simulink model "QuadRotor2Arm"  (R2019b)
(part 3 of 15)

  Revolute64 : sm_lib/Joints/Revolute Joint  JointMode=Normal  SenseConstraintForce=off  SenseConstraintForceX=off  SenseConstraintForceY=off  SenseConstraintForceZ=off  SenseConstraintTorque=off  SenseConstraintTorqueX=off  SenseConstraintTorqueY=off  SenseConstraintTorqueZ=off  SenseTotalForce=off  SenseTotalForceX=off  SenseTotalForceY=off  SenseTotalForceZ=off  SenseTotalTorque=off  SenseTotalTorqueX=off  SenseTotalTorqueY=off  SenseTotalTorqueZ=off  CompositeWrenchDir=FollowerOnBase  CompositeWrenchFrame=BaseFrame  EquilibriumPosition=0  EquilibriumPositionUnits=rad  SpringStiffness=0  SpringStiffnessUnits=N*m/rad  DampingCoefficient=0  DampingCoefficientUnits=N*m/(rad/s)  TorqueActuationMode=NoTorque  MotionActuationMode=ComputedMotion  SensePosition=off  SenseVelocity=off  SenseAcceleration=off  SenseTorqueForce=off  SenseLowerLimitTorqueForce=off  SenseUpperLimitTorqueForce=off  LowerLimitSpecify=off  LowerLimitBound=-90  LowerLimitBoundUnits=deg  LowerLimitStiffness=1e4  LowerLimitStiffnessUnits=N*m/deg  LowerLimitDamping=10  LowerLimitDampingUnits=N*m/(deg/s)  LowerLimitTransitionRegionWidth=0.1  LowerLimitTransitionRegionWidthUnits=deg  UpperLimitSpecify=off  UpperLimitBound=90  UpperLimitBoundUnits=deg  UpperLimitStiffness=1e4  UpperLimitStiffnessUnits=N*m/deg  UpperLimitDamping=10  UpperLimitDampingUnits=N*m/(deg/s)  UpperLimitTransitionRegionWidth=0.1  UpperLimitTransitionRegionWidthUnits=deg  PositionTargetSpecify=on  PositionTargetPriority=Low  PositionTargetValue=smiData.RevoluteJoint(65).Rz.Pos  PositionTargetValueUnits=deg  VelocityTargetSpecify=off  VelocityTargetPriority=High  VelocityTargetValue=0  VelocityTargetValueUnits=deg/s
  Revolute65 : sm_lib/Joints/Revolute Joint  JointMode=Normal  SenseConstraintForce=off  SenseConstraintForceX=off  SenseConstraintForceY=off  SenseConstraintForceZ=off  SenseConstraintTorque=off  SenseConstraintTorqueX=off  SenseConstraintTorqueY=off  SenseConstraintTorqueZ=off  SenseTotalForce=off  SenseTotalForceX=off  SenseTotalForceY=off  SenseTotalForceZ=off  SenseTotalTorque=off  SenseTotalTorqueX=off  SenseTotalTorqueY=off  SenseTotalTorqueZ=off  CompositeWrenchDir=FollowerOnBase  CompositeWrenchFrame=BaseFrame  EquilibriumPosition=0  EquilibriumPositionUnits=rad  SpringStiffness=0  SpringStiffnessUnits=N*m/rad  DampingCoefficient=0  DampingCoefficientUnits=N*m/(rad/s)  TorqueActuationMode=NoTorque  MotionActuationMode=ComputedMotion  SensePosition=off  SenseVelocity=off  SenseAcceleration=off  SenseTorqueForce=off  SenseLowerLimitTorqueForce=off  SenseUpperLimitTorqueForce=off  LowerLimitSpecify=off  LowerLimitBound=-90  LowerLimitBoundUnits=deg  LowerLimitStiffness=1e4  LowerLimitStiffnessUnits=N*m/deg  LowerLimitDamping=10  LowerLimitDampingUnits=N*m/(deg/s)  LowerLimitTransitionRegionWidth=0.1  LowerLimitTransitionRegionWidthUnits=deg  UpperLimitSpecify=off  UpperLimitBound=90  UpperLimitBoundUnits=deg  UpperLimitStiffness=1e4  UpperLimitStiffnessUnits=N*m/deg  UpperLimitDamping=10  UpperLimitDampingUnits=N*m/(deg/s)  UpperLimitTransitionRegionWidth=0.1  UpperLimitTransitionRegionWidthUnits=deg  PositionTargetSpecify=on  PositionTargetPriority=Low  PositionTargetValue=smiData.RevoluteJoint(66).Rz.Pos  PositionTargetValueUnits=deg  VelocityTargetSpecify=off  VelocityTargetPriority=High  VelocityTargetValue=0  VelocityTargetValueUnits=deg/s
  Revolute66 : sm_lib/Joints/Revolute Joint  JointMode=Normal  SenseConstraintForce=off  SenseConstraintForceX=off  SenseConstraintForceY=off  SenseConstraintForceZ=off  SenseConstraintTorque=off  SenseConstraintTorqueX=off  SenseConstraintTorqueY=off  SenseConstraintTorqueZ=off  SenseTotalForce=off  SenseTotalForceX=off  SenseTotalForceY=off  SenseTotalForceZ=off  SenseTotalTorque=off  SenseTotalTorqueX=off  SenseTotalTorqueY=off  SenseTotalTorqueZ=off  CompositeWrenchDir=FollowerOnBase  CompositeWrenchFrame=BaseFrame  EquilibriumPosition=0  EquilibriumPositionUnits=rad  SpringStiffness=0  SpringStiffnessUnits=N*m/rad  DampingCoefficient=0  DampingCoefficientUnits=N*m/(rad/s)  TorqueActuationMode=NoTorque  MotionActuationMode=ComputedMotion  SensePosition=off  SenseVelocity=off  SenseAcceleration=off  SenseTorqueForce=off  SenseLowerLimitTorqueForce=off  SenseUpperLimitTorqueForce=off  LowerLimitSpecify=off  LowerLimitBound=-90  LowerLimitBoundUnits=deg  LowerLimitStiffness=1e4  LowerLimitStiffnessUnits=N*m/deg  LowerLimitDamping=10  LowerLimitDampingUnits=N*m/(deg/s)  LowerLimitTransitionRegionWidth=0.1  LowerLimitTransitionRegionWidthUnits=deg  UpperLimitSpecify=off  UpperLimitBound=90  UpperLimitBoundUnits=deg  UpperLimitStiffness=1e4  UpperLimitStiffnessUnits=N*m/deg  UpperLimitDamping=10  UpperLimitDampingUnits=N*m/(deg/s)  UpperLimitTransitionRegionWidth=0.1  UpperLimitTransitionRegionWidthUnits=deg  PositionTargetSpecify=on  PositionTargetPriority=Low  PositionTargetValue=smiData.RevoluteJoint(67).Rz.Pos  PositionTargetValueUnits=deg  VelocityTargetSpecify=off  VelocityTargetPriority=High  VelocityTargetValue=0  VelocityTargetValueUnits=deg/s
  Revolute67 : sm_lib/Joints/Revolute Joint  JointMode=Normal  SenseConstraintForce=off  SenseConstraintForceX=off  SenseConstraintForceY=off  SenseConstraintForceZ=off  SenseConstraintTorque=off  SenseConstraintTorqueX=off  SenseConstraintTorqueY=off  SenseConstraintTorqueZ=off  SenseTotalForce=off  SenseTotalForceX=off  SenseTotalForceY=off  SenseTotalForceZ=off  SenseTotalTorque=off  SenseTotalTorqueX=off  SenseTotalTorqueY=off  SenseTotalTorqueZ=off  CompositeWrenchDir=FollowerOnBase  CompositeWrenchFrame=BaseFrame  EquilibriumPosition=0  EquilibriumPositionUnits=rad  SpringStiffness=0  SpringStiffnessUnits=N*m/rad  DampingCoefficient=0  DampingCoefficientUnits=N*m/(rad/s)  TorqueActuationMode=NoTorque  MotionActuationMode=ComputedMotion  SensePosition=off  SenseVelocity=off  SenseAcceleration=off  SenseTorqueForce=off  SenseLowerLimitTorqueForce=off  SenseUpperLimitTorqueForce=off  LowerLimitSpecify=off  LowerLimitBound=-90  LowerLimitBoundUnits=deg  LowerLimitStiffness=1e4  LowerLimitStiffnessUnits=N*m/deg  LowerLimitDamping=10  LowerLimitDampingUnits=N*m/(deg/s)  LowerLimitTransitionRegionWidth=0.1  LowerLimitTransitionRegionWidthUnits=deg  UpperLimitSpecify=off  UpperLimitBound=90  UpperLimitBoundUnits=deg  UpperLimitStiffness=1e4  UpperLimitStiffnessUnits=N*m/deg  UpperLimitDamping=10  UpperLimitDampingUnits=N*m/(deg/s)  UpperLimitTransitionRegionWidth=0.1  UpperLimitTransitionRegionWidthUnits=deg  PositionTargetSpecify=on  PositionTargetPriority=Low  PositionTargetValue=smiData.RevoluteJoint(68).Rz.Pos  PositionTargetValueUnits=deg  VelocityTargetSpecify=off  VelocityTargetPriority=High  VelocityTargetValue=0  VelocityTargetValueUnits=deg/s
  Revolute68 : sm_lib/Joints/Revolute Joint  JointMode=Normal  SenseConstraintForce=off  SenseConstraintForceX=off  SenseConstraintForceY=off  SenseConstraintForceZ=off  SenseConstraintTorque=off  SenseConstraintTorqueX=off  SenseConstraintTorqueY=off  SenseConstraintTorqueZ=off  SenseTotalForce=off  SenseTotalForceX=off  SenseTotalForceY=off  SenseTotalForceZ=off  SenseTotalTorque=off  SenseTotalTorqueX=off  SenseTotalTorqueY=off  SenseTotalTorqueZ=off  CompositeWrenchDir=FollowerOnBase  CompositeWrenchFrame=BaseFrame  EquilibriumPosition=0  EquilibriumPositionUnits=rad  SpringStiffness=0  SpringStiffnessUnits=N*m/rad  DampingCoefficient=0  DampingCoefficientUnits=N*m/(rad/s)  TorqueActuationMode=NoTorque  MotionActuationMode=ComputedMotion  SensePosition=off  SenseVelocity=off  SenseAcceleration=off  SenseTorqueForce=off  SenseLowerLimitTorqueForce=off  SenseUpperLimitTorqueForce=off  LowerLimitSpecify=off  LowerLimitBound=-90  LowerLimitBoundUnits=deg  LowerLimitStiffness=1e4  LowerLimitStiffnessUnits=N*m/deg  LowerLimitDamping=10  LowerLimitDampingUnits=N*m/(deg/s)  LowerLimitTransitionRegionWidth=0.1  LowerLimitTransitionRegionWidthUnits=deg  UpperLimitSpecify=off  UpperLimitBound=90  UpperLimitBoundUnits=deg  UpperLimitStiffness=1e4  UpperLimitStiffnessUnits=N*m/deg  UpperLimitDamping=10  UpperLimitDampingUnits=N*m/(deg/s)  UpperLimitTransitionRegionWidth=0.1  UpperLimitTransitionRegionWidthUnits=deg  PositionTargetSpecify=on  PositionTargetPriority=Low  PositionTargetValue=smiData.RevoluteJoint(69).Rz.Pos  PositionTargetValueUnits=deg  VelocityTargetSpecify=off  VelocityTargetPriority=High  VelocityTargetValue=0  VelocityTargetValueUnits=deg/s
  Revolute69 : sm_lib/Joints/Revolute Joint  JointMode=Normal  SenseConstraintForce=off  SenseConstraintForceX=off  SenseConstraintForceY=off  SenseConstraintForceZ=off  SenseConstraintTorque=off  SenseConstraintTorqueX=off  SenseConstraintTorqueY=off  SenseConstraintTorqueZ=off  SenseTotalForce=off  SenseTotalForceX=off  SenseTotalForceY=off  SenseTotalForceZ=off  SenseTotalTorque=off  SenseTotalTorqueX=off  SenseTotalTorqueY=off  SenseTotalTorqueZ=off  CompositeWrenchDir=FollowerOnBase  CompositeWrenchFrame=BaseFrame  EquilibriumPosition=0  EquilibriumPositionUnits=rad  SpringStiffness=0  SpringStiffnessUnits=N*m/rad  DampingCoefficient=0  DampingCoefficientUnits=N*m/(rad/s)  TorqueActuationMode=NoTorque  MotionActuationMode=ComputedMotion  SensePosition=off  SenseVelocity=off  SenseAcceleration=off  SenseTorqueForce=off  SenseLowerLimitTorqueForce=off  SenseUpperLimitTorqueForce=off  LowerLimitSpecify=off  LowerLimitBound=-90  LowerLimitBoundUnits=deg  LowerLimitStiffness=1e4  LowerLimitStiffnessUnits=N*m/deg  LowerLimitDamping=10  LowerLimitDampingUnits=N*m/(deg/s)  LowerLimitTransitionRegionWidth=0.1  LowerLimitTransitionRegionWidthUnits=deg  UpperLimitSpecify=off  UpperLimitBound=90  UpperLimitBoundUnits=deg  UpperLimitStiffness=1e4  UpperLimitStiffnessUnits=N*m/deg  UpperLimitDamping=10  UpperLimitDampingUnits=N*m/(deg/s)  UpperLimitTransitionRegionWidth=0.1  UpperLimitTransitionRegionWidthUnits=deg  PositionTargetSpecify=on  PositionTargetPriority=Low  PositionTargetValue=smiData.RevoluteJoint(70).Rz.Pos  PositionTargetValueUnits=deg  VelocityTargetSpecify=off  VelocityTargetPriority=High  VelocityTargetValue=0  VelocityTargetValueUnits=deg/s
  Revolute7 : sm_lib/Joints/Revolute Joint  JointMode=Normal  SenseConstraintForce=off  SenseConstraintForceX=off  SenseConstraintForceY=off  SenseConstraintForceZ=off  SenseConstraintTorque=off  SenseConstraintTorqueX=off  SenseConstraintTorqueY=off  SenseConstraintTorqueZ=off  SenseTotalForce=off  SenseTotalForceX=off  SenseTotalForceY=off  SenseTotalForceZ=off  SenseTotalTorque=off  SenseTotalTorqueX=off  SenseTotalTorqueY=off  SenseTotalTorqueZ=off  CompositeWrenchDir=FollowerOnBase  CompositeWrenchFrame=BaseFrame  EquilibriumPosition=0  EquilibriumPositionUnits=rad  SpringStiffness=0  SpringStiffnessUnits=N*m/rad  DampingCoefficient=0  DampingCoefficientUnits=N*m/(rad/s)  TorqueActuationMode=NoTorque  MotionActuationMode=ComputedMotion  SensePosition=off  SenseVelocity=off  SenseAcceleration=off  SenseTorqueForce=off  SenseLowerLimitTorqueForce=off  SenseUpperLimitTorqueForce=off  LowerLimitSpecify=off  LowerLimitBound=-90  LowerLimitBoundUnits=deg  LowerLimitStiffness=1e4  LowerLimitStiffnessUnits=N*m/deg  LowerLimitDamping=10  LowerLimitDampingUnits=N*m/(deg/s)  LowerLimitTransitionRegionWidth=0.1  LowerLimitTransitionRegionWidthUnits=deg  UpperLimitSpecify=off  UpperLimitBound=90  UpperLimitBoundUnits=deg  UpperLimitStiffness=1e4  UpperLimitStiffnessUnits=N*m/deg  UpperLimitDamping=10  UpperLimitDampingUnits=N*m/(deg/s)  UpperLimitTransitionRegionWidth=0.1  UpperLimitTransitionRegionWidthUnits=deg  PositionTargetSpecify=on  PositionTargetPriority=Low  PositionTargetValue=smiData.RevoluteJoint(8).Rz.Pos  PositionTargetValueUnits=deg  VelocityTargetSpecify=off  VelocityTargetPriority=High  VelocityTargetValue=0  VelocityTargetValueUnits=deg/s
  Revolute70 : sm_lib/Joints/Revolute Joint  JointMode=Normal  SenseConstraintForce=off  SenseConstraintForceX=off  SenseConstraintForceY=off  SenseConstraintForceZ=off  SenseConstraintTorque=off  SenseConstraintTorqueX=off  SenseConstraintTorqueY=off  SenseConstraintTorqueZ=off  SenseTotalForce=off  SenseTotalForceX=off  SenseTotalForceY=off  SenseTotalForceZ=off  SenseTotalTorque=off  SenseTotalTorqueX=off  SenseTotalTorqueY=off  SenseTotalTorqueZ=off  CompositeWrenchDir=FollowerOnBase  CompositeWrenchFrame=BaseFrame  EquilibriumPosition=0  EquilibriumPositionUnits=rad  SpringStiffness=0  SpringStiffnessUnits=N*m/rad  DampingCoefficient=0  DampingCoefficientUnits=N*m/(rad/s)  TorqueActuationMode=NoTorque  MotionActuationMode=ComputedMotion  SensePosition=off  SenseVelocity=off  SenseAcceleration=off  SenseTorqueForce=off  SenseLowerLimitTorqueForce=off  SenseUpperLimitTorqueForce=off  LowerLimitSpecify=off  LowerLimitBound=-90  LowerLimitBoundUnits=deg  LowerLimitStiffness=1e4  LowerLimitStiffnessUnits=N*m/deg  LowerLimitDamping=10  LowerLimitDampingUnits=N*m/(deg/s)  LowerLimitTransitionRegionWidth=0.1  LowerLimitTransitionRegionWidthUnits=deg  UpperLimitSpecify=off  UpperLimitBound=90  UpperLimitBoundUnits=deg  UpperLimitStiffness=1e4  UpperLimitStiffnessUnits=N*m/deg  UpperLimitDamping=10  UpperLimitDampingUnits=N*m/(deg/s)  UpperLimitTransitionRegionWidth=0.1  UpperLimitTransitionRegionWidthUnits=deg  PositionTargetSpecify=on  PositionTargetPriority=Low  PositionTargetValue=smiData.RevoluteJoint(71).Rz.Pos  PositionTargetValueUnits=deg  VelocityTargetSpecify=off  VelocityTargetPriority=High  VelocityTargetValue=0  VelocityTargetValueUnits=deg/s
  Revolute71 : sm_lib/Joints/Revolute Joint  JointMode=Normal  SenseConstraintForce=off  SenseConstraintForceX=off  SenseConstraintForceY=off  SenseConstraintForceZ=off  SenseConstraintTorque=off  SenseConstraintTorqueX=off  SenseConstraintTorqueY=off  SenseConstraintTorqueZ=off  SenseTotalForce=off  SenseTotalForceX=off  SenseTotalForceY=off  SenseTotalForceZ=off  SenseTotalTorque=off  SenseTotalTorqueX=off  SenseTotalTorqueY=off  SenseTotalTorqueZ=off  CompositeWrenchDir=FollowerOnBase  CompositeWrenchFrame=BaseFrame  EquilibriumPosition=0  EquilibriumPositionUnits=rad  SpringStiffness=0  SpringStiffnessUnits=N*m/rad  DampingCoefficient=0  DampingCoefficientUnits=N*m/(rad/s)  TorqueActuationMode=NoTorque  MotionActuationMode=ComputedMotion  SensePosition=off  SenseVelocity=off  SenseAcceleration=off  SenseTorqueForce=off  SenseLowerLimitTorqueForce=off  SenseUpperLimitTorqueForce=off  LowerLimitSpecify=off  LowerLimitBound=-90  LowerLimitBoundUnits=deg  LowerLimitStiffness=1e4  LowerLimitStiffnessUnits=N*m/deg  LowerLimitDamping=10  LowerLimitDampingUnits=N*m/(deg/s)  LowerLimitTransitionRegionWidth=0.1  LowerLimitTransitionRegionWidthUnits=deg  UpperLimitSpecify=off  UpperLimitBound=90  UpperLimitBoundUnits=deg  UpperLimitStiffness=1e4  UpperLimitStiffnessUnits=N*m/deg  UpperLimitDamping=10  UpperLimitDampingUnits=N*m/(deg/s)  UpperLimitTransitionRegionWidth=0.1  UpperLimitTransitionRegionWidthUnits=deg  PositionTargetSpecify=on  PositionTargetPriority=Low  PositionTargetValue=smiData.RevoluteJoint(72).Rz.Pos  PositionTargetValueUnits=deg  VelocityTargetSpecify=off  VelocityTargetPriority=High  VelocityTargetValue=0  VelocityTargetValueUnits=deg/s
  Revolute72 : sm_lib/Joints/Revolute Joint  JointMode=Normal  SenseConstraintForce=off  SenseConstraintForceX=off  SenseConstraintForceY=off  SenseConstraintForceZ=off  SenseConstraintTorque=off  SenseConstraintTorqueX=off  SenseConstraintTorqueY=off  SenseConstraintTorqueZ=off  SenseTotalForce=off  SenseTotalForceX=off  SenseTotalForceY=off  SenseTotalForceZ=off  SenseTotalTorque=off  SenseTotalTorqueX=off  SenseTotalTorqueY=off  SenseTotalTorqueZ=off  CompositeWrenchDir=FollowerOnBase  CompositeWrenchFrame=BaseFrame  EquilibriumPosition=0  EquilibriumPositionUnits=rad  SpringStiffness=0  SpringStiffnessUnits=N*m/rad  DampingCoefficient=0  DampingCoefficientUnits=N*m/(rad/s)  TorqueActuationMode=NoTorque  MotionActuationMode=ComputedMotion  SensePosition=off  SenseVelocity=off  SenseAcceleration=off  SenseTorqueForce=off  SenseLowerLimitTorqueForce=off  SenseUpperLimitTorqueForce=off  LowerLimitSpecify=off  LowerLimitBound=-90  LowerLimitBoundUnits=deg  LowerLimitStiffness=1e4  LowerLimitStiffnessUnits=N*m/deg  LowerLimitDamping=10  LowerLimitDampingUnits=N*m/(deg/s)  LowerLimitTransitionRegionWidth=0.1  LowerLimitTransitionRegionWidthUnits=deg  UpperLimitSpecify=off  UpperLimitBound=90  UpperLimitBoundUnits=deg  UpperLimitStiffness=1e4  UpperLimitStiffnessUnits=N*m/deg  UpperLimitDamping=10  UpperLimitDampingUnits=N*m/(deg/s)  UpperLimitTransitionRegionWidth=0.1  UpperLimitTransitionRegionWidthUnits=deg  PositionTargetSpecify=on  PositionTargetPriority=Low  PositionTargetValue=smiData.RevoluteJoint(73).Rz.Pos  PositionTargetValueUnits=deg  VelocityTargetSpecify=off  VelocityTargetPriority=High  VelocityTargetValue=0  VelocityTargetValueUnits=deg/s
  Revolute73 : sm_lib/Joints/Revolute Joint  JointMode=Normal  SenseConstraintForce=off  SenseConstraintForceX=off  SenseConstraintForceY=off  SenseConstraintForceZ=off  SenseConstraintTorque=off  SenseConstraintTorqueX=off  SenseConstraintTorqueY=off  SenseConstraintTorqueZ=off  SenseTotalForce=off  SenseTotalForceX=off  SenseTotalForceY=off  SenseTotalForceZ=off  SenseTotalTorque=off  SenseTotalTorqueX=off  SenseTotalTorqueY=off  SenseTotalTorqueZ=off  CompositeWrenchDir=FollowerOnBase  CompositeWrenchFrame=BaseFrame  EquilibriumPosition=0  EquilibriumPositionUnits=rad  SpringStiffness=0  SpringStiffnessUnits=N*m/rad  DampingCoefficient=0  DampingCoefficientUnits=N*m/(rad/s)  TorqueActuationMode=NoTorque  MotionActuationMode=ComputedMotion  SensePosition=off  SenseVelocity=off  SenseAcceleration=off  SenseTorqueForce=off  SenseLowerLimitTorqueForce=off  SenseUpperLimitTorqueForce=off  LowerLimitSpecify=off  LowerLimitBound=-90  LowerLimitBoundUnits=deg  LowerLimitStiffness=1e4  LowerLimitStiffnessUnits=N*m/deg  LowerLimitDamping=10  LowerLimitDampingUnits=N*m/(deg/s)  LowerLimitTransitionRegionWidth=0.1  LowerLimitTransitionRegionWidthUnits=deg  UpperLimitSpecify=off  UpperLimitBound=90  UpperLimitBoundUnits=deg  UpperLimitStiffness=1e4  UpperLimitStiffnessUnits=N*m/deg  UpperLimitDamping=10  UpperLimitDampingUnits=N*m/(deg/s)  UpperLimitTransitionRegionWidth=0.1  UpperLimitTransitionRegionWidthUnits=deg  PositionTargetSpecify=on  PositionTargetPriority=Low  PositionTargetValue=smiData.RevoluteJoint(74).Rz.Pos  PositionTargetValueUnits=deg  VelocityTargetSpecify=off  VelocityTargetPriority=High  VelocityTargetValue=0  VelocityTargetValueUnits=deg/s
  Revolute74 : sm_lib/Joints/Revolute Joint  JointMode=Normal  SenseConstraintForce=off  SenseConstraintForceX=off  SenseConstraintForceY=off  SenseConstraintForceZ=off  SenseConstraintTorque=off  SenseConstraintTorqueX=off  SenseConstraintTorqueY=off  SenseConstraintTorqueZ=off  SenseTotalForce=off  SenseTotalForceX=off  SenseTotalForceY=off  SenseTotalForceZ=off  SenseTotalTorque=off  SenseTotalTorqueX=off  SenseTotalTorqueY=off  SenseTotalTorqueZ=off  CompositeWrenchDir=FollowerOnBase  CompositeWrenchFrame=BaseFrame  EquilibriumPosition=0  EquilibriumPositionUnits=rad  SpringStiffness=0  SpringStiffnessUnits=N*m/rad  DampingCoefficient=0  DampingCoefficientUnits=N*m/(rad/s)  TorqueActuationMode=NoTorque  MotionActuationMode=ComputedMotion  SensePosition=off  SenseVelocity=off  SenseAcceleration=off  SenseTorqueForce=off  SenseLowerLimitTorqueForce=off  SenseUpperLimitTorqueForce=off  LowerLimitSpecify=off  LowerLimitBound=-90  LowerLimitBoundUnits=deg  LowerLimitStiffness=1e4  LowerLimitStiffnessUnits=N*m/deg  LowerLimitDamping=10  LowerLimitDampingUnits=N*m/(deg/s)  LowerLimitTransitionRegionWidth=0.1  LowerLimitTransitionRegionWidthUnits=deg  UpperLimitSpecify=off  UpperLimitBound=90  UpperLimitBoundUnits=deg  UpperLimitStiffness=1e4  UpperLimitStiffnessUnits=N*m/deg  UpperLimitDamping=10  UpperLimitDampingUnits=N*m/(deg/s)  UpperLimitTransitionRegionWidth=0.1  UpperLimitTransitionRegionWidthUnits=deg  PositionTargetSpecify=on  PositionTargetPriority=Low  PositionTargetValue=smiData.RevoluteJoint(75).Rz.Pos  PositionTargetValueUnits=deg  VelocityTargetSpecify=off  VelocityTargetPriority=High  VelocityTargetValue=0  VelocityTargetValueUnits=deg/s
  Revolute75 : sm_lib/Joints/Revolute Joint  JointMode=Normal  SenseConstraintForce=off  SenseConstraintForceX=off  SenseConstraintForceY=off  SenseConstraintForceZ=off  SenseConstraintTorque=off  SenseConstraintTorqueX=off  SenseConstraintTorqueY=off  SenseConstraintTorqueZ=off  SenseTotalForce=off  SenseTotalForceX=off  SenseTotalForceY=off  SenseTotalForceZ=off  SenseTotalTorque=off  SenseTotalTorqueX=off  SenseTotalTorqueY=off  SenseTotalTorqueZ=off  CompositeWrenchDir=FollowerOnBase  CompositeWrenchFrame=BaseFrame  EquilibriumPosition=0  EquilibriumPositionUnits=rad  SpringStiffness=0  SpringStiffnessUnits=N*m/rad  DampingCoefficient=0  DampingCoefficientUnits=N*m/(rad/s)  TorqueActuationMode=NoTorque  MotionActuationMode=ComputedMotion  SensePosition=off  SenseVelocity=off  SenseAcceleration=off  SenseTorqueForce=off  SenseLowerLimitTorqueForce=off  SenseUpperLimitTorqueForce=off  LowerLimitSpecify=off  LowerLimitBound=-90  LowerLimitBoundUnits=deg  LowerLimitStiffness=1e4  LowerLimitStiffnessUnits=N*m/deg  LowerLimitDamping=10  LowerLimitDampingUnits=N*m/(deg/s)  LowerLimitTransitionRegionWidth=0.1  LowerLimitTransitionRegionWidthUnits=deg  UpperLimitSpecify=off  UpperLimitBound=90  UpperLimitBoundUnits=deg  UpperLimitStiffness=1e4  UpperLimitStiffnessUnits=N*m/deg  UpperLimitDamping=10  UpperLimitDampingUnits=N*m/(deg/s)  UpperLimitTransitionRegionWidth=0.1  UpperLimitTransitionRegionWidthUnits=deg  PositionTargetSpecify=on  PositionTargetPriority=Low  PositionTargetValue=smiData.RevoluteJoint(76).Rz.Pos  PositionTargetValueUnits=deg  VelocityTargetSpecify=off  VelocityTargetPriority=High  VelocityTargetValue=0  VelocityTargetValueUnits=deg/s
  Revolute76 : sm_lib/Joints/Revolute Joint  JointMode=Normal  SenseConstraintForce=off  SenseConstraintForceX=off  SenseConstraintForceY=off  SenseConstraintForceZ=off  SenseConstraintTorque=off  SenseConstraintTorqueX=off  SenseConstraintTorqueY=off  SenseConstraintTorqueZ=off  SenseTotalForce=off  SenseTotalForceX=off  SenseTotalForceY=off  SenseTotalForceZ=off  SenseTotalTorque=off  SenseTotalTorqueX=off  SenseTotalTorqueY=off  SenseTotalTorqueZ=off  CompositeWrenchDir=FollowerOnBase  CompositeWrenchFrame=BaseFrame  EquilibriumPosition=0  EquilibriumPositionUnits=rad  SpringStiffness=0  SpringStiffnessUnits=N*m/rad  DampingCoefficient=0  DampingCoefficientUnits=N*m/(rad/s)  TorqueActuationMode=NoTorque  MotionActuationMode=ComputedMotion  SensePosition=off  SenseVelocity=off  SenseAcceleration=off  SenseTorqueForce=off  SenseLowerLimitTorqueForce=off  SenseUpperLimitTorqueForce=off  LowerLimitSpecify=off  LowerLimitBound=-90  LowerLimitBoundUnits=deg  LowerLimitStiffness=1e4  LowerLimitStiffnessUnits=N*m/deg  LowerLimitDamping=10  LowerLimitDampingUnits=N*m/(deg/s)  LowerLimitTransitionRegionWidth=0.1  LowerLimitTransitionRegionWidthUnits=deg  UpperLimitSpecify=off  UpperLimitBound=90  UpperLimitBoundUnits=deg  UpperLimitStiffness=1e4  UpperLimitStiffnessUnits=N*m/deg  UpperLimitDamping=10  UpperLimitDampingUnits=N*m/(deg/s)  UpperLimitTransitionRegionWidth=0.1  UpperLimitTransitionRegionWidthUnits=deg  PositionTargetSpecify=on  PositionTargetPriority=Low  PositionTargetValue=smiData.RevoluteJoint(77).Rz.Pos  PositionTargetValueUnits=deg  VelocityTargetSpecify=off  VelocityTargetPriority=High  VelocityTargetValue=0  VelocityTargetValueUnits=deg/s
  Revolute77 : sm_lib/Joints/Revolute Joint  JointMode=Normal  SenseConstraintForce=off  SenseConstraintForceX=off  SenseConstraintForceY=off  SenseConstraintForceZ=off  SenseConstraintTorque=off  SenseConstraintTorqueX=off  SenseConstraintTorqueY=off  SenseConstraintTorqueZ=off  SenseTotalForce=off  SenseTotalForceX=off  SenseTotalForceY=off  SenseTotalForceZ=off  SenseTotalTorque=off  SenseTotalTorqueX=off  SenseTotalTorqueY=off  SenseTotalTorqueZ=off  CompositeWrenchDir=FollowerOnBase  CompositeWrenchFrame=BaseFrame  EquilibriumPosition=0  EquilibriumPositionUnits=rad  SpringStiffness=0  SpringStiffnessUnits=N*m/rad  DampingCoefficient=0  DampingCoefficientUnits=N*m/(rad/s)  TorqueActuationMode=NoTorque  MotionActuationMode=ComputedMotion  SensePosition=off  SenseVelocity=off  SenseAcceleration=off  SenseTorqueForce=off  SenseLowerLimitTorqueForce=off  SenseUpperLimitTorqueForce=off  LowerLimitSpecify=off  LowerLimitBound=-90  LowerLimitBoundUnits=deg  LowerLimitStiffness=1e4  LowerLimitStiffnessUnits=N*m/deg  LowerLimitDamping=10  LowerLimitDampingUnits=N*m/(deg/s)  LowerLimitTransitionRegionWidth=0.1  LowerLimitTransitionRegionWidthUnits=deg  UpperLimitSpecify=off  UpperLimitBound=90  UpperLimitBoundUnits=deg  UpperLimitStiffness=1e4  UpperLimitStiffnessUnits=N*m/deg  UpperLimitDamping=10  UpperLimitDampingUnits=N*m/(deg/s)  UpperLimitTransitionRegionWidth=0.1  UpperLimitTransitionRegionWidthUnits=deg  PositionTargetSpecify=on  PositionTargetPriority=Low  PositionTargetValue=smiData.RevoluteJoint(78).Rz.Pos  PositionTargetValueUnits=deg  VelocityTargetSpecify=off  VelocityTargetPriority=High  VelocityTargetValue=0  VelocityTargetValueUnits=deg/s
  Revolute78 : sm_lib/Joints/Revolute Joint  JointMode=Normal  SenseConstraintForce=off  SenseConstraintForceX=off  SenseConstraintForceY=off  SenseConstraintForceZ=off  SenseConstraintTorque=off  SenseConstraintTorqueX=off  SenseConstraintTorqueY=off  SenseConstraintTorqueZ=off  SenseTotalForce=off  SenseTotalForceX=off  SenseTotalForceY=off  SenseTotalForceZ=off  SenseTotalTorque=off  SenseTotalTorqueX=off  SenseTotalTorqueY=off  SenseTotalTorqueZ=off  CompositeWrenchDir=FollowerOnBase  CompositeWrenchFrame=BaseFrame  EquilibriumPosition=0  EquilibriumPositionUnits=rad  SpringStiffness=0  SpringStiffnessUnits=N*m/rad  DampingCoefficient=0  DampingCoefficientUnits=N*m/(rad/s)  TorqueActuationMode=NoTorque  MotionActuationMode=ComputedMotion  SensePosition=off  SenseVelocity=off  SenseAcceleration=off  SenseTorqueForce=off  SenseLowerLimitTorqueForce=off  SenseUpperLimitTorqueForce=off  LowerLimitSpecify=off  LowerLimitBound=-90  LowerLimitBoundUnits=deg  LowerLimitStiffness=1e4  LowerLimitStiffnessUnits=N*m/deg  LowerLimitDamping=10  LowerLimitDampingUnits=N*m/(deg/s)  LowerLimitTransitionRegionWidth=0.1  LowerLimitTransitionRegionWidthUnits=deg  UpperLimitSpecify=off  UpperLimitBound=90  UpperLimitBoundUnits=deg  UpperLimitStiffness=1e4  UpperLimitStiffnessUnits=N*m/deg  UpperLimitDamping=10  UpperLimitDampingUnits=N*m/(deg/s)  UpperLimitTransitionRegionWidth=0.1  UpperLimitTransitionRegionWidthUnits=deg  PositionTargetSpecify=on  PositionTargetPriority=Low  PositionTargetValue=smiData.RevoluteJoint(79).Rz.Pos  PositionTargetValueUnits=deg  VelocityTargetSpecify=off  VelocityTargetPriority=High  VelocityTargetValue=0  VelocityTargetValueUnits=deg/s
  Revolute79 : sm_lib/Joints/Revolute Joint  JointMode=Normal  SenseConstraintForce=off  SenseConstraintForceX=off  SenseConstraintForceY=off  SenseConstraintForceZ=off  SenseConstraintTorque=off  SenseConstraintTorqueX=off  SenseConstraintTorqueY=off  SenseConstraintTorqueZ=off  SenseTotalForce=off  SenseTotalForceX=off  SenseTotalForceY=off  SenseTotalForceZ=off  SenseTotalTorque=off  SenseTotalTorqueX=off  SenseTotalTorqueY=off  SenseTotalTorqueZ=off  CompositeWrenchDir=FollowerOnBase  CompositeWrenchFrame=BaseFrame  EquilibriumPosition=0  EquilibriumPositionUnits=rad  SpringStiffness=0  SpringStiffnessUnits=N*m/rad  DampingCoefficient=0  DampingCoefficientUnits=N*m/(rad/s)  TorqueActuationMode=NoTorque  MotionActuationMode=ComputedMotion  SensePosition=off  SenseVelocity=off  SenseAcceleration=off  SenseTorqueForce=off  SenseLowerLimitTorqueForce=off  SenseUpperLimitTorqueForce=off  LowerLimitSpecify=off  LowerLimitBound=-90  LowerLimitBoundUnits=deg  LowerLimitStiffness=1e4  LowerLimitStiffnessUnits=N*m/deg  LowerLimitDamping=10  LowerLimitDampingUnits=N*m/(deg/s)  LowerLimitTransitionRegionWidth=0.1  LowerLimitTransitionRegionWidthUnits=deg  UpperLimitSpecify=off  UpperLimitBound=90  UpperLimitBoundUnits=deg  UpperLimitStiffness=1e4  UpperLimitStiffnessUnits=N*m/deg  UpperLimitDamping=10  UpperLimitDampingUnits=N*m/(deg/s)  UpperLimitTransitionRegionWidth=0.1  UpperLimitTransitionRegionWidthUnits=deg  PositionTargetSpecify=on  PositionTargetPriority=Low  PositionTargetValue=smiData.RevoluteJoint(80).Rz.Pos  PositionTargetValueUnits=deg  VelocityTargetSpecify=off  VelocityTargetPriority=High  VelocityTargetValue=0  VelocityTargetValueUnits=deg/s
  Revolute8 : sm_lib/Joints/Revolute Joint  JointMode=Normal  SenseConstraintForce=off  SenseConstraintForceX=off  SenseConstraintForceY=off  SenseConstraintForceZ=off  SenseConstraintTorque=off  SenseConstraintTorqueX=off  SenseConstraintTorqueY=off  SenseConstraintTorqueZ=off  SenseTotalForce=off  SenseTotalForceX=off  SenseTotalForceY=off  SenseTotalForceZ=off  SenseTotalTorque=off  SenseTotalTorqueX=off  SenseTotalTorqueY=off  SenseTotalTorqueZ=off  CompositeWrenchDir=FollowerOnBase  CompositeWrenchFrame=BaseFrame  EquilibriumPosition=0  EquilibriumPositionUnits=rad  SpringStiffness=0  SpringStiffnessUnits=N*m/rad  DampingCoefficient=0  DampingCoefficientUnits=N*m/(rad/s)  TorqueActuationMode=NoTorque  MotionActuationMode=ComputedMotion  SensePosition=off  SenseVelocity=off  SenseAcceleration=off  SenseTorqueForce=off  SenseLowerLimitTorqueForce=off  SenseUpperLimitTorqueForce=off  LowerLimitSpecify=off  LowerLimitBound=-90  LowerLimitBoundUnits=deg  LowerLimitStiffness=1e4  LowerLimitStiffnessUnits=N*m/deg  LowerLimitDamping=10  LowerLimitDampingUnits=N*m/(deg/s)  LowerLimitTransitionRegionWidth=0.1  LowerLimitTransitionRegionWidthUnits=deg  UpperLimitSpecify=off  UpperLimitBound=90  UpperLimitBoundUnits=deg  UpperLimitStiffness=1e4  UpperLimitStiffnessUnits=N*m/deg  UpperLimitDamping=10  UpperLimitDampingUnits=N*m/(deg/s)  UpperLimitTransitionRegionWidth=0.1  UpperLimitTransitionRegionWidthUnits=deg  PositionTargetSpecify=on  PositionTargetPriority=Low  PositionTargetValue=smiData.RevoluteJoint(9).Rz.Pos  PositionTargetValueUnits=deg  VelocityTargetSpecify=off  VelocityTargetPriority=High  VelocityTargetValue=0  VelocityTargetValueUnits=deg/s
  Revolute80 : sm_lib/Joints/Revolute Joint  JointMode=Normal  SenseConstraintForce=off  SenseConstraintForceX=off  SenseConstraintForceY=off  SenseConstraintForceZ=off  SenseConstraintTorque=off  SenseConstraintTorqueX=off  SenseConstraintTorqueY=off  SenseConstraintTorqueZ=off  SenseTotalForce=off  SenseTotalForceX=off  SenseTotalForceY=off  SenseTotalForceZ=off  SenseTotalTorque=off  SenseTotalTorqueX=off  SenseTotalTorqueY=off  SenseTotalTorqueZ=off  CompositeWrenchDir=FollowerOnBase  CompositeWrenchFrame=BaseFrame  EquilibriumPosition=0  EquilibriumPositionUnits=rad  SpringStiffness=0  SpringStiffnessUnits=N*m/rad  DampingCoefficient=0  DampingCoefficientUnits=N*m/(rad/s)  TorqueActuationMode=NoTorque  MotionActuationMode=ComputedMotion  SensePosition=off  SenseVelocity=off  SenseAcceleration=off  SenseTorqueForce=off  SenseLowerLimitTorqueForce=off  SenseUpperLimitTorqueForce=off  LowerLimitSpecify=off  LowerLimitBound=-90  LowerLimitBoundUnits=deg  LowerLimitStiffness=1e4  LowerLimitStiffnessUnits=N*m/deg  LowerLimitDamping=10  LowerLimitDampingUnits=N*m/(deg/s)  LowerLimitTransitionRegionWidth=0.1  LowerLimitTransitionRegionWidthUnits=deg  UpperLimitSpecify=off  UpperLimitBound=90  UpperLimitBoundUnits=deg  UpperLimitStiffness=1e4  UpperLimitStiffnessUnits=N*m/deg  UpperLimitDamping=10  UpperLimitDampingUnits=N*m/(deg/s)  UpperLimitTransitionRegionWidth=0.1  UpperLimitTransitionRegionWidthUnits=deg  PositionTargetSpecify=on  PositionTargetPriority=Low  PositionTargetValue=smiData.RevoluteJoint(81).Rz.Pos  PositionTargetValueUnits=deg  VelocityTargetSpecify=off  VelocityTargetPriority=High  VelocityTargetValue=0  VelocityTargetValueUnits=deg/s
  Revolute9 : sm_lib/Joints/Revolute Joint  JointMode=Normal  SenseConstraintForce=off  SenseConstraintForceX=off  SenseConstraintForceY=off  SenseConstraintForceZ=off  SenseConstraintTorque=off  SenseConstraintTorqueX=off  SenseConstraintTorqueY=off  SenseConstraintTorqueZ=off  SenseTotalForce=off  SenseTotalForceX=off  SenseTotalForceY=off  SenseTotalForceZ=off  SenseTotalTorque=off  SenseTotalTorqueX=off  SenseTotalTorqueY=off  SenseTotalTorqueZ=off  CompositeWrenchDir=FollowerOnBase  CompositeWrenchFrame=BaseFrame  EquilibriumPosition=0  EquilibriumPositionUnits=rad  SpringStiffness=0  SpringStiffnessUnits=N*m/rad  DampingCoefficient=0  DampingCoefficientUnits=N*m/(rad/s)  TorqueActuationMode=NoTorque  MotionActuationMode=ComputedMotion  SensePosition=off  SenseVelocity=off  SenseAcceleration=off  SenseTorqueForce=off  SenseLowerLimitTorqueForce=off  SenseUpperLimitTorqueForce=off  LowerLimitSpecify=off  LowerLimitBound=-90  LowerLimitBoundUnits=deg  LowerLimitStiffness=1e4  LowerLimitStiffnessUnits=N*m/deg  LowerLimitDamping=10  LowerLimitDampingUnits=N*m/(deg/s)  LowerLimitTransitionRegionWidth=0.1  LowerLimitTransitionRegionWidthUnits=deg  UpperLimitSpecify=off  UpperLimitBound=90  UpperLimitBoundUnits=deg  UpperLimitStiffness=1e4  UpperLimitStiffnessUnits=N*m/deg  UpperLimitDamping=10  UpperLimitDampingUnits=N*m/(deg/s)  UpperLimitTransitionRegionWidth=0.1  UpperLimitTransitionRegionWidthUnits=deg  PositionTargetSpecify=on  PositionTargetPriority=Low  PositionTargetValue=smiData.RevoluteJoint(10).Rz.Pos  PositionTargetValueUnits=deg  VelocityTargetSpecify=off  VelocityTargetPriority=High  VelocityTargetValue=0  VelocityTargetValueUnits=deg/s
  Solver Configuration : nesl_utility/Solver Configuration  PhysicalDomain=network_engine_domain  SubClassName=solver  LeftPortType=input  RightPortType=generic  Tones=[]  Harmonics=[]  SimulateNoise=off  Profile=off  UseLocalSampling=off  EnableSwitchedLinearOptims=on  FrequencyDomain=off  UseCCode=off  RelTol=0.001  AbsTol=1e-06  MinStep=1e-09  ToWorkspace=off  RevertToSquareIcSolve=off  NumHomotopyIterations=100  PhasorMode=off  PhasorModeNumHarmonics=1  DoDC=off  ResidualTolerance=1e-09  UseLocalSolver=off  LocalSolverChoice=NE_BACKWARD_EULER_ADVANCER  LocalSolverSampleTime=0.001  DoFixedCost=off  MaxNonlinIter=3  MaxModeIter=2  LinearAlgebra=auto  EquationFormulation=NE_TIME_EF  DelaysMemoryBudget=1024  AutomaticFiltering=on  FilteringTimeConstant=0.001  PartitionStorageMethod=AS_NEEDED  PartitionMemoryBudget=1024  PartitionMethod=ROBUST
  Spektrum_AR6110_1_RIGID : Subsystem
  Transform : sm_lib/Frames and Transforms/Rigid Transform  TranslationMethod=Cartesian  TranslationStandardOffset=0  TranslationLengthUnit=mm  TranslationStandardAxis=+Z  TranslationCartesianOffset=smiData.RigidTransform(407).translation  TranslationROffset=0  TranslationROffsetUnits=m  TranslationZOffset=0  TranslationZOffsetUnits=m  TranslationThetaOffset=0  TranslationThetaOffsetUnits=deg  RotationMethod=ArbitraryAxis  RotationAngleUnits=rad  RotationStandardAxis=+Z  RotationAngle=smiData.RigidTransform(407).angle  RotationArbitraryAxis=smiData.RigidTransform(407).axis  FollAlignAxisA=+X  BaseAlignAxisA=+Y  FollAlignAxisB=+Y  BaseAlignAxisB=+Z  RotationSequenceAxes=FollowerAxes  RotationSequence=XYX  RotationSequenceAngles=[0 0 0]  RotationSequenceAnglesUnits=deg  RotationMatrix=[1 0 0; 0 1 0; 0 0 1]
  Transform1 : sm_lib/Frames and Transforms/Rigid Transform  TranslationMethod=Cartesian  TranslationStandardOffset=0  TranslationLengthUnit=mm  TranslationStandardAxis=+Z  TranslationCartesianOffset=smiData.RigidTransform(408).translation  TranslationROffset=0  TranslationROffsetUnits=m  TranslationZOffset=0  TranslationZOffsetUnits=m  TranslationThetaOffset=0  TranslationThetaOffsetUnits=deg  RotationMethod=ArbitraryAxis  RotationAngleUnits=rad  RotationStandardAxis=+Z  RotationAngle=smiData.RigidTransform(408).angle  RotationArbitraryAxis=smiData.RigidTransform(408).axis  FollAlignAxisA=+X  BaseAlignAxisA=+Y  FollAlignAxisB=+Y  BaseAlignAxisB=+Z  RotationSequenceAxes=FollowerAxes  RotationSequence=XYX  RotationSequenceAngles=[0 0 0]  RotationSequenceAnglesUnits=deg  RotationMatrix=[1 0 0; 0 1 0; 0 0 1]
  Turnigy_18_11_2000kv_Micro_Brushless_Outrunner_1_RIGID : Subsystem
  Turnigy_18_11_2000kv_Micro_Brushless_Outrunner_2_RIGID : Subsystem
  Turnigy_18_11_2000kv_Micro_Brushless_Outrunner_3_RIGID : Subsystem
  Turnigy_18_11_2000kv_Micro_Brushless_Outrunner_4_RIGID : Subsystem
  Turnigy_NanoTech_850mah_2S_Lipo_1_RIGID : Subsystem
  Turnigy_Plush_6A_Speed_Controller_1_RIGID : Subsystem
  Turnigy_Plush_6A_Speed_Controller_2_RIGID : Subsystem
  Turnigy_Plush_6A_Speed_Controller_3_RIGID : Subsystem
  Turnigy_Plush_6A_Speed_Controller_4_RIGID : Subsystem
  World : sm_lib/Frames and Transforms/World Frame
  de_1_RIGID : Subsystem
  hex_nut_style_1_gradeab_din_10_RIGID : Subsystem
  hex_nut_style_1_gradeab_din_11_RIGID : Subsystem
  hex_nut_style_1_gradeab_din_12_RIGID : Subsystem
  hex_nut_style_1_gradeab_din_13_RIGID : Subsystem
  hex_nut_style_1_gradeab_din_15_RIGID : Subsystem
  hex_nut_style_1_gradeab_din_16_RIGID : Subsystem
  hex_nut_style_1_gradeab_din_17_RIGID : Subsystem
  hex_nut_style_1_gradeab_din_1_RIGID : Subsystem
  hex_nut_style_1_gradeab_din_2_RIGID : Subsystem
  hex_nut_style_1_gradeab_din_3_RIGID : Subsystem
  hex_nut_style_1_gradeab_din_4_RIGID : Subsystem
  hex_nut_style_1_gradeab_din_5_RIGID : Subsystem
  hex_nut_style_1_gradeab_din_6_RIGID : Subsystem
  hex_nut_style_1_gradeab_din_7_RIGID : Subsystem
  hex_nut_style_1_gradeab_din_8_RIGID : Subsystem
  hex_nut_style_1_gradeab_din_9_RIGID : Subsystem
  socket_head_cap_screw_din_10_RIGID : Subsystem
  socket_head_cap_screw_din_11_RIGID : Subsystem
  socket_head_cap_screw_din_12_RIGID : Subsystem
  socket_head_cap_screw_din_13_RIGID : Subsystem
  socket_head_cap_screw_din_14_RIGID : Subsystem
  socket_head_cap_screw_din_15_RIGID : Subsystem
  socket_head_cap_screw_din_16_RIGID : Subsystem
  socket_head_cap_screw_din_17_RIGID : Subsystem
  socket_head_cap_screw_din_18_RIGID : Subsystem
  socket_head_cap_screw_din_19_RIGID : Subsystem
  socket_head_cap_screw_din_1_RIGID : Subsystem
  socket_head_cap_screw_din_20_RIGID : Subsystem
  socket_head_cap_screw_din_21_RIGID : Subsystem
  socket_head_cap_screw_din_22_RIGID : Subsystem
  socket_head_cap_screw_din_23_RIGID : Subsystem
  socket_head_cap_screw_din_24_RIGID : Subsystem
  socket_head_cap_screw_din_25_RIGID : Subsystem
  socket_head_cap_screw_din_26_RIGID : Subsystem
  socket_head_cap_screw_din_27_RIGID : Subsystem
  socket_head_cap_screw_din_28_RIGID : Subsystem
  socket_head_cap_screw_din_29_RIGID : Subsystem
  socket_head_cap_screw_din_2_RIGID : Subsystem
  socket_head_cap_screw_din_30_RIGID : Subsystem
  socket_head_cap_screw_din_31_RIGID : Subsystem
  socket_head_cap_screw_din_32_RIGID : Subsystem
  socket_head_cap_screw_din_33_RIGID : Subsystem
  socket_head_cap_screw_din_34_RIGID : Subsystem
  socket_head_cap_screw_din_35_RIGID : Subsystem
  socket_head_cap_screw_din_36_RIGID : Subsystem
  socket_head_cap_screw_din_37_RIGID : Subsystem
  socket_head_cap_screw_din_38_RIGID : Subsystem
  socket_head_cap_screw_din_39_RIGID : Subsystem
  socket_head_cap_screw_din_3_RIGID : Subsystem
  socket_head_cap_screw_din_41_RIGID : Subsystem
  socket_head_cap_screw_din_42_RIGID : Subsystem
  socket_head_cap_screw_din_43_RIGID : Subsystem
  socket_head_cap_screw_din_44_RIGID : Subsystem
  socket_head_cap_screw_din_45_RIGID : Subsystem
  socket_head_cap_screw_din_46_RIGID : Subsystem
  socket_head_cap_screw_din_47_RIGID : Subsystem
  socket_head_cap_screw_din_48_RIGID : Subsystem
  socket_head_cap_screw_din_49_RIGID : Subsystem
  socket_head_cap_screw_din_4_RIGID : Subsystem
  socket_head_cap_screw_din_50_RIGID : Subsystem
  socket_head_cap_screw_din_51_RIGID : Subsystem
  socket_head_cap_screw_din_52_RIGID : Subsystem
  socket_head_cap_screw_din_53_RIGID : Subsystem
  socket_head_cap_screw_din_54_RIGID : Subsystem
  socket_head_cap_screw_din_55_RIGID : Subsystem
  socket_head_cap_screw_din_56_RIGID : Subsystem
  socket_head_cap_screw_din_57_RIGID : Subsystem
  socket_head_cap_screw_din_5_RIGID : Subsystem
  socket_head_cap_screw_din_6_RIGID : Subsystem
  socket_head_cap_screw_din_7_RIGID : Subsystem
  socket_head_cap_screw_din_8_RIGID : Subsystem
  socket_head_cap_screw_din_9_RIGID : Subsystem
  tay_1_1_RIGID : Subsystem
  tay_2_1_RIGID : Subsystem
  tay_han_1_RIGID : Subsystem
  x5x3L_Propeller_3_RIGID : Subsystem
  x5x3L_Propeller_4_RIGID : Subsystem
  x5x3R_Propeller_1_RIGID : Subsystem
  x5x3R_Propeller_2_RIGID : Subsystem
  connections:
  Transform/LConn1 -- MechanismConfiguration/RConn1 -- Solver Configuration/RConn1 -- World/RConn1 -- Transform1/LConn1
  Rectangular/LConn1 -- x5x3L_Propeller_3_RIGID/RConn2
  Cylindrical1/RConn1 -- x5x3L_Propeller_4_RIGID/LConn1
  Revolute26/RConn1 -- hex_nut_style_1_gradeab_din_3_RIGID/LConn1
  Revolute27/LConn1 -- Turnigy_18_11_2000kv_Micro_Brushless_Outrunner_1_RIGID/RConn4
  Revolute27/RConn1 -- hex_nut_style_1_gradeab_din_4_RIGID/LConn1
  Revolute28/LConn1 -- Turnigy_18_11_2000kv_Micro_Brushless_Outrunner_4_RIGID/RConn5
  Revolute28/RConn1 -- hex_nut_style_1_gradeab_din_5_RIGID/LConn1
  Revolute29/LConn1 -- Turnigy_18_11_2000kv_Micro_Brushless_Outrunner_4_RIGID/RConn3
  Revolute29/RConn1 -- hex_nut_style_1_gradeab_din_6_RIGID/LConn1
  Revolute30/LConn1 -- Turnigy_18_11_2000kv_Micro_Brushless_Outrunner_4_RIGID/RConn2
  Revolute30/RConn1 -- hex_nut_style_1_gradeab_din_7_RIGID/LConn1
  Revolute31/LConn1 -- Turnigy_18_11_2000kv_Micro_Brushless_Outrunner_4_RIGID/RConn1
  Rectangular1/LConn1 -- Turnigy_Plush_6A_Speed_Controller_1_RIGID/RConn2
  Revolute31/RConn1 -- hex_nut_style_1_gradeab_din_8_RIGID/LConn1
  Revolute32/LConn1 -- Turnigy_18_11_2000kv_Micro_Brushless_Outrunner_3_RIGID/RConn4
  Revolute32/RConn1 -- hex_nut_style_1_gradeab_din_9_RIGID/LConn1
  Revolute33/LConn1 -- Turnigy_18_11_2000kv_Micro_Brushless_Outrunner_3_RIGID/RConn3
  Revolute33/RConn1 -- hex_nut_style_1_gradeab_din_10_RIGID/LConn1
  Revolute34/LConn1 -- Turnigy_18_11_2000kv_Micro_Brushless_Outrunner_3_RIGID/RConn2
  Revolute34/RConn1 -- hex_nut_style_1_gradeab_din_11_RIGID/LConn1
  Revolute35/LConn1 -- Turnigy_18_11_2000kv_Micro_Brushless_Outrunner_3_RIGID/RConn1
  Revolute35/RConn1 -- hex_nut_style_1_gradeab_din_12_RIGID/LConn1
  Revolute36/LConn1 -- Turnigy_18_11_2000kv_Micro_Brushless_Outrunner_2_RIGID/RConn6
  Rectangular1/RConn1 -- Turnigy_Plush_6A_Speed_Controller_2_RIGID/LConn1
  Revolute36/RConn1 -- hex_nut_style_1_gradeab_din_13_RIGID/LConn1
  Revolute37/LConn1 -- Turnigy_18_11_2000kv_Micro_Brushless_Outrunner_2_RIGID/RConn5
  Revolute37/RConn1 -- hex_nut_style_1_gradeab_din_15_RIGID/LConn1
  Revolute38/LConn1 -- Turnigy_18_11_2000kv_Micro_Brushless_Outrunner_2_RIGID/RConn4
  Revolute38/RConn1 -- hex_nut_style_1_gradeab_din_16_RIGID/LConn1
  Revolute39/LConn1 -- Turnigy_18_11_2000kv_Micro_Brushless_Outrunner_2_RIGID/RConn3
  Revolute39/RConn1 -- hex_nut_style_1_gradeab_din_17_RIGID/LConn1
  QRM005_Top_Frame_Ring_1_RIGID/RConn15 -- Revolute40/LConn1
  QRM103_Frame_Spacer_15mm_1_RIGID/LConn1 -- Revolute40/RConn1
  Cylindrical9/LConn1 -- QRM005_Top_Frame_Ring_1_RIGID/RConn16
  Prismatic/LConn1 -- Turnigy_Plush_6A_Speed_Controller_1_RIGID/RConn1
  Cylindrical9/RConn1 -- QRM103_Frame_Spacer_15mm_2_RIGID/LConn2
  Cylindrical10/LConn1 -- QRM005_Top_Frame_Ring_1_RIGID/RConn13
  Cylindrical10/RConn1 -- QRM103_Frame_Spacer_15mm_3_RIGID/LConn1
  Cylindrical11/LConn1 -- QRM005_Top_Frame_Ring_1_RIGID/RConn11
  Cylindrical11/RConn1 -- QRM103_Frame_Spacer_15mm_4_RIGID/LConn1
  QRM005_Top_Frame_Ring_1_RIGID/RConn7 -- Revolute41/LConn1
  Revolute41/RConn1 -- socket_head_cap_screw_din_29_RIGID/LConn1
  QRM005_Top_Frame_Ring_1_RIGID/RConn6 -- Revolute42/LConn1
  Revolute42/RConn1 -- socket_head_cap_screw_din_30_RIGID/LConn1
  QRM005_Top_Frame_Ring_1_RIGID/RConn4 -- Revolute43/LConn1
  Prismatic/RConn1 -- Turnigy_Plush_6A_Speed_Controller_4_RIGID/LConn1
  Revolute43/RConn1 -- socket_head_cap_screw_din_31_RIGID/LConn1
  QRM005_Top_Frame_Ring_1_RIGID/RConn3 -- Revolute44/LConn1
  Revolute44/RConn1 -- socket_head_cap_screw_din_32_RIGID/LConn1
  QRM005_Top_Frame_Ring_1_RIGID/RConn2 -- Revolute45/LConn1
  Revolute45/RConn1 -- socket_head_cap_screw_din_33_RIGID/LConn1
  QRM005_Top_Frame_Ring_1_RIGID/RConn1 -- Revolute46/LConn1
  Revolute46/RConn1 -- socket_head_cap_screw_din_34_RIGID/LConn1
  QRM005_Top_Frame_Ring_1_RIGID/RConn14 -- Revolute47/LConn1
  Revolute47/RConn1 -- socket_head_cap_screw_din_35_RIGID/LConn1
  QRM005_Top_Frame_Ring_1_RIGID/RConn12 -- Revolute48/LConn1
  Prismatic1/LConn1 -- Turnigy_Plush_6A_Speed_Controller_2_RIGID/RConn1
  Revolute48/RConn1 -- socket_head_cap_screw_din_36_RIGID/LConn1
  Revolute49/LConn1 -- tay_1_1_RIGID/RConn1
  Revolute49/RConn1 -- tay_2_1_RIGID/LConn2
  tay_2_1_RIGID/LConn1 -- tay_han_1_RIGID/LConn1
  Parallel/LConn1 -- QRM004_Bottom_Frame_Ring_1_RIGID/RConn5
  Parallel/RConn1 -- de_1_RIGID/LConn1
  Revolute50/LConn1 -- de_1_RIGID/RConn1
  Revolute50/RConn1 -- tay_1_1_RIGID/LConn1
  Prismatic3/LConn1 -- QRM003_Battery_Tray_1_RIGID/RConn2
  Prismatic3/RConn1 -- Turnigy_NanoTech_850mah_2S_Lipo_1_RIGID/LConn1
  Prismatic1/RConn1 -- Turnigy_Plush_6A_Speed_Controller_3_RIGID/LConn1
  QRM003_Battery_Tray_1_RIGID/RConn1 -- Revolute51/LConn1
  Revolute51/RConn1 -- socket_head_cap_screw_din_10_RIGID/LConn1
  Cylindrical12/LConn1 -- QRM005_Top_Frame_Ring_1_RIGID/RConn10
  Cylindrical12/RConn1 -- QRM101_Frame_Spacer_5mm_1_RIGID/LConn1
  Planar9/LConn1 -- QRM101_Frame_Spacer_5mm_1_RIGID/RConn1
  Planar9/RConn1 -- QRM101_Frame_Spacer_5mm_3_RIGID/LConn3
  Planar10/LConn1 -- QRM101_Frame_Spacer_5mm_1_RIGID/RConn2
  Planar10/RConn1 -- QRM101_Frame_Spacer_5mm_4_RIGID/LConn2
  QRM101_Frame_Spacer_5mm_2_RIGID/RConn2 -- Revolute52/LConn1
  HobbyKing_Multi_Rotor_Control_Board_1_RIGID/LConn2 -- Revolute52/RConn1
  HobbyKing_Multi_Rotor_Control_Board_1_RIGID/RConn4 -- Revolute/LConn1
  Cylindrical13/LConn1 -- QRM005_Top_Frame_Ring_1_RIGID/RConn8
  Cylindrical13/RConn1 -- QRM101_Frame_Spacer_5mm_2_RIGID/LConn1
  Planar11/LConn1 -- QRM101_Frame_Spacer_5mm_2_RIGID/RConn1
  Planar11/RConn1 -- QRM101_Frame_Spacer_5mm_3_RIGID/LConn2
  Cylindrical14/LConn1 -- QRM101_Frame_Spacer_5mm_3_RIGID/RConn1
  Cylindrical14/RConn1 -- HobbyKing_Multi_Rotor_Control_Board_1_RIGID/LConn1
  Cylindrical15/LConn1 -- QRM005_Top_Frame_Ring_1_RIGID/RConn5
  Cylindrical15/RConn1 -- QRM101_Frame_Spacer_5mm_3_RIGID/LConn1
  QRM005_Top_Frame_Ring_1_RIGID/RConn9 -- Revolute53/LConn1
  QRM101_Frame_Spacer_5mm_4_RIGID/LConn1 -- Revolute53/RConn1
  Revolute/RConn1 -- socket_head_cap_screw_din_37_RIGID/LConn1
  QRM103_Frame_Spacer_15mm_3_RIGID/RConn2 -- Revolute54/LConn1
  QRM006_Electronic_Cover_1_RIGID/LConn2 -- Revolute54/RConn1
  Cylindrical16/LConn1 -- QRM103_Frame_Spacer_15mm_4_RIGID/RConn1
  Cylindrical16/RConn1 -- QRM006_Electronic_Cover_1_RIGID/LConn1
  Planar12/LConn1 -- QRM103_Frame_Spacer_15mm_1_RIGID/RConn2
  Planar12/RConn1 -- QRM103_Frame_Spacer_15mm_2_RIGID/LConn1
  Planar13/LConn1 -- QRM103_Frame_Spacer_15mm_1_RIGID/RConn1
  Planar13/RConn1 -- QRM103_Frame_Spacer_15mm_3_RIGID/LConn2
  Planar14/LConn1 -- QRM103_Frame_Spacer_15mm_3_RIGID/RConn1
  Planar14/RConn1 -- QRM103_Frame_Spacer_15mm_4_RIGID/LConn2
  HobbyKing_Multi_Rotor_Control_Board_1_RIGID/RConn3 -- Revolute1/LConn1
  Parallel1/LConn1 -- x5x3R_Propeller_1_RIGID/RConn1
  Parallel1/RConn1 -- x5x3R_Propeller_2_RIGID/LConn2
  Revolute55/LConn1 -- Turnigy_18_11_2000kv_Micro_Brushless_Outrunner_4_RIGID/RConn4
  Revolute55/RConn1 -- x5x3R_Propeller_1_RIGID/LConn1
  Cylindrical17/LConn1 -- Turnigy_18_11_2000kv_Micro_Brushless_Outrunner_2_RIGID/RConn2
  Cylindrical17/RConn1 -- x5x3R_Propeller_2_RIGID/LConn1
  Planar15/LConn1 -- Turnigy_18_11_2000kv_Micro_Brushless_Outrunner_1_RIGID/RConn3
  Planar15/RConn1 -- Turnigy_18_11_2000kv_Micro_Brushless_Outrunner_2_RIGID/LConn2
  Planar16/LConn1 -- Turnigy_18_11_2000kv_Micro_Brushless_Outrunner_1_RIGID/RConn2
  Planar16/RConn1 -- Turnigy_18_11_2000kv_Micro_Brushless_Outrunner_3_RIGID/LConn2
  Rectangular/RConn1 -- x5x3L_Propeller_4_RIGID/LConn2
  Revolute1/RConn1 -- socket_head_cap_screw_din_38_RIGID/LConn1
  Planar17/LConn1 -- Turnigy_18_11_2000kv_Micro_Brushless_Outrunner_1_RIGID/RConn1
  Planar17/RConn1 -- Turnigy_18_11_2000kv_Micro_Brushless_Outrunner_4_RIGID/LConn3
  Planar18/LConn1 -- Turnigy_18_11_2000kv_Micro_Brushless_Outrunner_2_RIGID/RConn1
  Planar18/RConn1 -- Turnigy_18_11_2000kv_Micro_Brushless_Outrunner_4_RIGID/LConn2
  Planar19/LConn1 -- QRM104_Threaded_Frame_Spacer_10mm_30_RIGID/RConn2
  Planar19/RConn1 -- QRM104_Threaded_Frame_Spacer_10mm_33_RIGID/LConn1
  Planar20/LConn1 -- QRM104_Threaded_Frame_Spacer_10mm_30_RIGID/RConn1
  Planar20/RConn1 -- QRM104_Threaded_Frame_Spacer_10mm_34_RIGID/LConn2
  Cylindrical18/LConn1 -- QRM001_Bottom_Arm_4_RIGID/RConn11
  Cylindrical18/RConn1 -- QRM104_Threaded_Frame_Spacer_10mm_30_RIGID/LConn1
  HobbyKing_Multi_Rotor_Control_Board_1_RIGID/RConn2 -- Revolute2/LConn1
  Planar21/LConn1 -- QRM104_Threaded_Frame_Spacer_10mm_33_RIGID/RConn1
  Planar21/RConn1 -- QRM104_Threaded_Frame_Spacer_10mm_38_RIGID/LConn1
  Cylindrical19/LConn1 -- QRM001_Bottom_Arm_3_RIGID/RConn11
  Cylindrical19/RConn1 -- QRM104_Threaded_Frame_Spacer_10mm_33_RIGID/LConn2
  Planar22/LConn1 -- QRM104_Threaded_Frame_Spacer_10mm_34_RIGID/RConn1
  Planar22/RConn1 -- QRM104_Threaded_Frame_Spacer_10mm_36_RIGID/LConn1
  Cylindrical20/LConn1 -- QRM001_Bottom_Arm_4_RIGID/RConn8
  Cylindrical20/RConn1 -- QRM104_Threaded_Frame_Spacer_10mm_34_RIGID/LConn1
  Planar23/LConn1 -- QRM104_Threaded_Frame_Spacer_10mm_35_RIGID/RConn1
  Planar23/RConn1 -- QRM104_Threaded_Frame_Spacer_10mm_39_RIGID/LConn3
  Revolute2/RConn1 -- socket_head_cap_screw_din_39_RIGID/LConn1
  Cylindrical21/LConn1 -- QRM001_Bottom_Arm_3_RIGID/RConn10
  Cylindrical21/RConn1 -- QRM104_Threaded_Frame_Spacer_10mm_35_RIGID/LConn1
  Planar24/LConn1 -- QRM104_Threaded_Frame_Spacer_10mm_36_RIGID/RConn1
  Planar24/RConn1 -- QRM104_Threaded_Frame_Spacer_10mm_37_RIGID/LConn1
  Cylindrical22/LConn1 -- QRM001_Bottom_Arm_1_RIGID/RConn2
  Cylindrical22/RConn1 -- QRM104_Threaded_Frame_Spacer_10mm_36_RIGID/LConn2
  QRM001_Bottom_Arm_2_RIGID/RConn11 -- Revolute56/LConn1
  QRM104_Threaded_Frame_Spacer_10mm_37_RIGID/LConn2 -- Revolute56/RConn1
  Planar25/LConn1 -- QRM104_Threaded_Frame_Spacer_10mm_38_RIGID/RConn1
  Planar25/RConn1 -- QRM104_Threaded_Frame_Spacer_10mm_39_RIGID/LConn2
  HobbyKing_Multi_Rotor_Control_Board_1_RIGID/RConn1 -- Revolute3/LConn1
  Cylindrical23/LConn1 -- QRM001_Bottom_Arm_1_RIGID/RConn10
  Cylindrical23/RConn1 -- QRM104_Threaded_Frame_Spacer_10mm_38_RIGID/LConn2
  Cylindrical24/LConn1 -- QRM001_Bottom_Arm_2_RIGID/RConn12
  Cylindrical24/RConn1 -- QRM104_Threaded_Frame_Spacer_10mm_39_RIGID/LConn1
  Planar26/LConn1 -- QRM104_Threaded_Frame_Spacer_10mm_40_RIGID/RConn1
  Planar26/RConn1 -- QRM002_Top_Arm_2_RIGID/LConn3
  Cylindrical25/LConn1 -- QRM102_Frame_Spacer_10mm_2_RIGID/RConn4
  Cylindrical25/RConn1 -- QRM104_Threaded_Frame_Spacer_10mm_40_RIGID/LConn1
  Planar27/LConn1 -- QRM104_Threaded_Frame_Spacer_10mm_40_RIGID/RConn4
  Planar27/RConn1 -- QRM104_Threaded_Frame_Spacer_10mm_43_RIGID/LConn2
  Revolute3/RConn1 -- socket_head_cap_screw_din_41_RIGID/LConn1
  Planar28/LConn1 -- QRM104_Threaded_Frame_Spacer_10mm_40_RIGID/RConn2
  Planar28/RConn1 -- QRM104_Threaded_Frame_Spacer_10mm_45_RIGID/LConn3
  Cylindrical26/LConn1 -- QRM104_Threaded_Frame_Spacer_10mm_40_RIGID/RConn3
  Cylindrical26/RConn1 -- QRM102_Frame_Spacer_10mm_25_RIGID/LConn2
  Planar29/LConn1 -- QRM104_Threaded_Frame_Spacer_10mm_41_RIGID/RConn3
  Planar29/RConn1 -- QRM002_Top_Arm_1_RIGID/LConn3
  Cylindrical27/LConn1 -- QRM102_Frame_Spacer_10mm_1_RIGID/RConn4
  Cylindrical27/RConn1 -- QRM104_Threaded_Frame_Spacer_10mm_41_RIGID/LConn1
  Planar30/LConn1 -- QRM104_Threaded_Frame_Spacer_10mm_41_RIGID/RConn1
  Planar30/RConn1 -- QRM104_Threaded_Frame_Spacer_10mm_45_RIGID/LConn4
  QRM002_Top_Arm_1_RIGID/RConn2 -- Revolute4/LConn1
  Cylindrical28/LConn1 -- QRM104_Threaded_Frame_Spacer_10mm_41_RIGID/RConn2
  Cylindrical28/RConn1 -- QRM102_Frame_Spacer_10mm_27_RIGID/LConn2
  Cylindrical29/LConn1 -- QRM102_Frame_Spacer_10mm_3_RIGID/RConn3
  Cylindrical29/RConn1 -- QRM104_Threaded_Frame_Spacer_10mm_42_RIGID/LConn1
  Planar31/LConn1 -- QRM104_Threaded_Frame_Spacer_10mm_42_RIGID/RConn1
  Planar31/RConn1 -- QRM104_Threaded_Frame_Spacer_10mm_43_RIGID/LConn3
  Cylindrical30/LConn1 -- QRM104_Threaded_Frame_Spacer_10mm_42_RIGID/RConn2
  Cylindrical30/RConn1 -- QRM102_Frame_Spacer_10mm_30_RIGID/LConn3
  Cylindrical31/LConn1 -- QRM104_Threaded_Frame_Spacer_10mm_43_RIGID/RConn1
  Cylindrical31/RConn1 -- QRM002_Top_Arm_1_RIGID/LConn2
  Revolute4/RConn1 -- socket_head_cap_screw_din_7_RIGID/LConn1
  Cylindrical32/LConn1 -- QRM102_Frame_Spacer_10mm_5_RIGID/RConn4
  Cylindrical32/RConn1 -- QRM104_Threaded_Frame_Spacer_10mm_43_RIGID/LConn1
  Cylindrical33/LConn1 -- QRM104_Threaded_Frame_Spacer_10mm_43_RIGID/RConn2
  Cylindrical33/RConn1 -- QRM102_Frame_Spacer_10mm_26_RIGID/LConn1
  Cylindrical34/LConn1 -- QRM102_Frame_Spacer_10mm_6_RIGID/RConn2
  Cylindrical34/RConn1 -- QRM104_Threaded_Frame_Spacer_10mm_44_RIGID/LConn2
  Planar32/LConn1 -- QRM104_Threaded_Frame_Spacer_10mm_44_RIGID/RConn1
  Planar32/RConn1 -- QRM003_Battery_Tray_1_RIGID/LConn3
  Planar33/LConn1 -- QRM104_Threaded_Frame_Spacer_10mm_44_RIGID/RConn4
  Planar33/RConn1 -- QRM104_Threaded_Frame_Spacer_10mm_45_RIGID/LConn2
  QRM002_Top_Arm_1_RIGID/RConn1 -- Revolute5/LConn1
  Planar34/LConn1 -- QRM104_Threaded_Frame_Spacer_10mm_44_RIGID/RConn2
  Planar34/RConn1 -- QRM104_Threaded_Frame_Spacer_10mm_46_RIGID/LConn2
  Planar35/LConn1 -- QRM001_Bottom_Arm_2_RIGID/RConn10
  Planar35/RConn1 -- QRM104_Threaded_Frame_Spacer_10mm_44_RIGID/LConn1
  Cylindrical35/LConn1 -- QRM104_Threaded_Frame_Spacer_10mm_44_RIGID/RConn3
  Cylindrical35/RConn1 -- QRM102_Frame_Spacer_10mm_29_RIGID/LConn1
  Cylindrical36/LConn1 -- QRM102_Frame_Spacer_10mm_7_RIGID/RConn3
  Cylindrical36/RConn1 -- QRM104_Threaded_Frame_Spacer_10mm_45_RIGID/LConn1
  Planar36/LConn1 -- QRM104_Threaded_Frame_Spacer_10mm_45_RIGID/RConn2
  Planar36/RConn1 -- QRM104_Threaded_Frame_Spacer_10mm_47_RIGID/LConn2
  Revolute5/RConn1 -- socket_head_cap_screw_din_8_RIGID/LConn1
  Cylindrical37/LConn1 -- QRM104_Threaded_Frame_Spacer_10mm_45_RIGID/RConn1
  Cylindrical37/RConn1 -- QRM102_Frame_Spacer_10mm_31_RIGID/LConn1
  Cylindrical38/LConn1 -- QRM104_Threaded_Frame_Spacer_10mm_46_RIGID/RConn1
  Cylindrical38/RConn1 -- QRM002_Top_Arm_2_RIGID/LConn2
  Cylindrical39/LConn1 -- QRM102_Frame_Spacer_10mm_8_RIGID/RConn2
  Cylindrical39/RConn1 -- QRM104_Threaded_Frame_Spacer_10mm_46_RIGID/LConn1
  Cylindrical40/LConn1 -- QRM104_Threaded_Frame_Spacer_10mm_46_RIGID/RConn2
  Cylindrical40/RConn1 -- QRM102_Frame_Spacer_10mm_28_RIGID/LConn1
  Cylindrical41/LConn1 -- QRM102_Frame_Spacer_10mm_4_RIGID/RConn2
  Cylindrical41/RConn1 -- QRM104_Threaded_Frame_Spacer_10mm_47_RIGID/LConn1
  QRM002_Top_Arm_2_RIGID/RConn2 -- Revolute6/LConn1
  Cylindrical42/LConn1 -- QRM001_Bottom_Arm_1_RIGID/RConn11
  Cylindrical42/RConn1 -- QRM002_Top_Arm_1_RIGID/LConn1
  Cylindrical43/LConn1 -- QRM102_Frame_Spacer_10mm_2_RIGID/RConn1
  Cylindrical43/RConn1 -- QRM001_Bottom_Arm_1_RIGID/LConn2
  Cylindrical44/LConn1 -- QRM102_Frame_Spacer_10mm_5_RIGID/RConn3
  Cylindrical44/RConn1 -- QRM001_Bottom_Arm_1_RIGID/LConn1
  Prismatic4/LConn1 -- QRM001_Bottom_Arm_1_RIGID/RConn7
  Prismatic4/RConn1 -- Turnigy_18_11_2000kv_Micro_Brushless_Outrunner_1_RIGID/LConn1
  QRM001_Bottom_Arm_1_RIGID/RConn6 -- Revolute57/LConn1
  Revolute57/RConn1 -- socket_head_cap_screw_din_13_RIGID/LConn1
  Planar/LConn1 -- x5x3L_Propeller_3_RIGID/RConn1
  Revolute6/RConn1 -- socket_head_cap_screw_din_11_RIGID/LConn1
  QRM001_Bottom_Arm_1_RIGID/RConn5 -- Revolute58/LConn1
  Revolute58/RConn1 -- socket_head_cap_screw_din_14_RIGID/LConn1
  QRM001_Bottom_Arm_1_RIGID/RConn4 -- Revolute59/LConn1
  Revolute59/RConn1 -- socket_head_cap_screw_din_50_RIGID/LConn1
  QRM001_Bottom_Arm_1_RIGID/RConn3 -- Revolute60/LConn1
  Revolute60/RConn1 -- socket_head_cap_screw_din_51_RIGID/LConn1
  QRM001_Bottom_Arm_1_RIGID/RConn9 -- Revolute61/LConn1
  Revolute61/RConn1 -- socket_head_cap_screw_din_52_RIGID/LConn1
  QRM001_Bottom_Arm_1_RIGID/RConn8 -- Revolute62/LConn1
  Revolute62/RConn1 -- socket_head_cap_screw_din_53_RIGID/LConn1
  QRM002_Top_Arm_2_RIGID/RConn1 -- Revolute7/LConn1
  Planar37/LConn1 -- QRM001_Bottom_Arm_1_RIGID/RConn1
  Planar37/RConn1 -- QRM001_Bottom_Arm_2_RIGID/LConn4
  Planar38/LConn1 -- QRM102_Frame_Spacer_10mm_5_RIGID/RConn1
  Planar38/RConn1 -- QRM001_Bottom_Arm_2_RIGID/LConn3
  Cylindrical45/LConn1 -- QRM102_Frame_Spacer_10mm_6_RIGID/RConn1
  Cylindrical45/RConn1 -- QRM001_Bottom_Arm_2_RIGID/LConn2
  Cylindrical46/LConn1 -- QRM102_Frame_Spacer_10mm_7_RIGID/RConn1
  Cylindrical46/RConn1 -- QRM001_Bottom_Arm_2_RIGID/LConn1
  Cylindrical47/LConn1 -- QRM001_Bottom_Arm_2_RIGID/RConn7
  Cylindrical47/RConn1 -- QRM003_Battery_Tray_1_RIGID/LConn1
  Revolute7/RConn1 -- socket_head_cap_screw_din_12_RIGID/LConn1
  Prismatic5/LConn1 -- QRM001_Bottom_Arm_2_RIGID/RConn2
  Prismatic5/RConn1 -- Turnigy_18_11_2000kv_Micro_Brushless_Outrunner_4_RIGID/LConn1
  QRM001_Bottom_Arm_2_RIGID/RConn1 -- Revolute63/LConn1
  Revolute63/RConn1 -- socket_head_cap_screw_din_15_RIGID/LConn1
  QRM001_Bottom_Arm_2_RIGID/RConn9 -- Revolute64/LConn1
  Revolute64/RConn1 -- socket_head_cap_screw_din_16_RIGID/LConn1
  QRM001_Bottom_Arm_2_RIGID/RConn8 -- Revolute65/LConn1
  Revolute65/RConn1 -- socket_head_cap_screw_din_46_RIGID/LConn1
  QRM001_Bottom_Arm_2_RIGID/RConn6 -- Revolute66/LConn1
  Revolute66/RConn1 -- socket_head_cap_screw_din_47_RIGID/LConn1
  Cylindrical2/LConn1 -- QRM004_Bottom_Frame_Ring_1_RIGID/RConn9
  QRM001_Bottom_Arm_2_RIGID/RConn5 -- Revolute67/LConn1
  Revolute67/RConn1 -- socket_head_cap_screw_din_48_RIGID/LConn1
  QRM001_Bottom_Arm_2_RIGID/RConn4 -- Revolute68/LConn1
  Revolute68/RConn1 -- socket_head_cap_screw_din_49_RIGID/LConn1
  Planar39/LConn1 -- QRM001_Bottom_Arm_2_RIGID/RConn3
  Planar39/RConn1 -- QRM001_Bottom_Arm_4_RIGID/LConn2
  Cylindrical48/LConn1 -- QRM102_Frame_Spacer_10mm_3_RIGID/RConn1
  Cylindrical48/RConn1 -- QRM001_Bottom_Arm_3_RIGID/LConn2
  Cylindrical49/LConn1 -- QRM102_Frame_Spacer_10mm_4_RIGID/RConn1
  Cylindrical49/RConn1 -- QRM001_Bottom_Arm_3_RIGID/LConn1
  Cylindrical2/RConn1 -- QRM102_Frame_Spacer_10mm_1_RIGID/LConn1
  Cylindrical50/LConn1 -- QRM001_Bottom_Arm_3_RIGID/RConn7
  Cylindrical50/RConn1 -- QRM003_Battery_Tray_1_RIGID/LConn2
  Prismatic6/LConn1 -- QRM001_Bottom_Arm_3_RIGID/RConn5
  Prismatic6/RConn1 -- Turnigy_18_11_2000kv_Micro_Brushless_Outrunner_2_RIGID/LConn3
  QRM001_Bottom_Arm_3_RIGID/RConn6 -- Revolute69/LConn1
  Revolute69/RConn1 -- socket_head_cap_screw_din_19_RIGID/LConn1
  QRM001_Bottom_Arm_3_RIGID/RConn4 -- Revolute70/LConn1
  Revolute70/RConn1 -- socket_head_cap_screw_din_20_RIGID/LConn1
  QRM001_Bottom_Arm_3_RIGID/RConn3 -- Revolute71/LConn1
  Revolute71/RConn1 -- socket_head_cap_screw_din_54_RIGID/LConn1
  Cylindrical3/LConn1 -- QRM004_Bottom_Frame_Ring_1_RIGID/RConn16
  QRM001_Bottom_Arm_3_RIGID/RConn2 -- Revolute72/LConn1
  Revolute72/RConn1 -- socket_head_cap_screw_din_55_RIGID/LConn1
  QRM001_Bottom_Arm_3_RIGID/RConn9 -- Revolute73/LConn1
  Revolute73/RConn1 -- socket_head_cap_screw_din_56_RIGID/LConn1
  QRM001_Bottom_Arm_3_RIGID/RConn8 -- Revolute74/LConn1
  Revolute74/RConn1 -- socket_head_cap_screw_din_57_RIGID/LConn1
  Planar40/LConn1 -- QRM001_Bottom_Arm_3_RIGID/RConn1
  Planar40/RConn1 -- QRM001_Bottom_Arm_4_RIGID/LConn4
  Planar41/LConn1 -- Turnigy_Plush_6A_Speed_Controller_1_RIGID/RConn3
  Planar41/RConn1 -- QRM001_Bottom_Arm_4_RIGID/LConn1
  Cylindrical3/RConn1 -- QRM102_Frame_Spacer_10mm_2_RIGID/LConn1
  Cylindrical51/LConn1 -- QRM001_Bottom_Arm_4_RIGID/RConn10
  Cylindrical51/RConn1 -- QRM002_Top_Arm_2_RIGID/LConn1
  Cylindrical52/LConn1 -- QRM102_Frame_Spacer_10mm_1_RIGID/RConn1
  Cylindrical52/RConn1 -- QRM001_Bottom_Arm_4_RIGID/LConn5
  Cylindrical53/LConn1 -- QRM102_Frame_Spacer_10mm_8_RIGID/RConn1
  Cylindrical53/RConn1 -- QRM001_Bottom_Arm_4_RIGID/LConn3
  Planar42/LConn1 -- QRM001_Bottom_Arm_4_RIGID/RConn9
  Planar42/RConn1 -- Turnigy_18_11_2000kv_Micro_Brushless_Outrunner_2_RIGID/LConn1
  Prismatic7/LConn1 -- QRM001_Bottom_Arm_4_RIGID/RConn2
  Prismatic7/RConn1 -- Turnigy_18_11_2000kv_Micro_Brushless_Outrunner_3_RIGID/LConn1
  Cylindrical4/LConn1 -- QRM004_Bottom_Frame_Ring_1_RIGID/RConn17
  QRM001_Bottom_Arm_4_RIGID/RConn7 -- Revolute75/LConn1
  Revolute75/RConn1 -- socket_head_cap_screw_din_17_RIGID/LConn1
  QRM001_Bottom_Arm_4_RIGID/RConn6 -- Revolute76/LConn1
  Revolute76/RConn1 -- socket_head_cap_screw_din_18_RIGID/LConn1
  QRM001_Bottom_Arm_4_RIGID/RConn5 -- Revolute77/LConn1
  Revolute77/RConn1 -- socket_head_cap_screw_din_42_RIGID/LConn1
  QRM001_Bottom_Arm_4_RIGID/RConn4 -- Revolute78/LConn1
  Revolute78/RConn1 -- socket_head_cap_screw_din_43_RIGID/LConn1
  QRM001_Bottom_Arm_4_RIGID/RConn3 -- Revolute79/LConn1
  Revolute79/RConn1 -- socket_head_cap_screw_din_44_RIGID/LConn1
  Cylindrical4/RConn1 -- QRM102_Frame_Spacer_10mm_3_RIGID/LConn2
  QRM001_Bottom_Arm_4_RIGID/RConn1 -- Revolute80/LConn1
  Revolute80/RConn1 -- socket_head_cap_screw_din_45_RIGID/LConn1
  Planar43/LConn1 -- QRM002_Top_Arm_2_RIGID/RConn3
  Planar43/RConn1 -- QRM102_Frame_Spacer_10mm_25_RIGID/LConn1
  Planar44/LConn1 -- QRM102_Frame_Spacer_10mm_25_RIGID/RConn1
  Planar44/RConn1 -- QRM102_Frame_Spacer_10mm_27_RIGID/LConn1
  Planar45/LConn1 -- QRM102_Frame_Spacer_10mm_26_RIGID/RConn1
  Planar45/RConn1 -- QRM102_Frame_Spacer_10mm_30_RIGID/LConn2
  Planar46/LConn1 -- QRM102_Frame_Spacer_10mm_27_RIGID/RConn1
  Planar46/RConn1 -- QRM102_Frame_Spacer_10mm_28_RIGID/LConn2
  Cylindrical5/LConn1 -- QRM004_Bottom_Frame_Ring_1_RIGID/RConn8
  Planar47/LConn1 -- QRM102_Frame_Spacer_10mm_28_RIGID/RConn1
  Planar47/RConn1 -- QRM102_Frame_Spacer_10mm_29_RIGID/LConn2
  Planar48/LConn1 -- QRM102_Frame_Spacer_10mm_29_RIGID/RConn2
  Planar48/RConn1 -- QRM102_Frame_Spacer_10mm_30_RIGID/LConn1
  Planar49/LConn1 -- QRM102_Frame_Spacer_10mm_29_RIGID/RConn1
  Planar49/RConn1 -- QRM102_Frame_Spacer_10mm_31_RIGID/LConn2
  Cylindrical54/LConn1 -- QRM102_Frame_Spacer_10mm_30_RIGID/RConn1
  Cylindrical54/RConn1 -- QRM005_Top_Frame_Ring_1_RIGID/LConn3
  Planar50/LConn1 -- QRM102_Frame_Spacer_10mm_31_RIGID/RConn2
  Planar50/RConn1 -- QRM005_Top_Frame_Ring_1_RIGID/LConn2
  Planar/RConn1 -- x5x3R_Propeller_1_RIGID/LConn2
  Cylindrical5/RConn1 -- QRM102_Frame_Spacer_10mm_4_RIGID/LConn1
  Planar51/LConn1 -- QRM102_Frame_Spacer_10mm_31_RIGID/RConn1
  Planar51/RConn1 -- QRM102_Frame_Spacer_10mm_32_RIGID/LConn2
  Cylindrical55/LConn1 -- QRM102_Frame_Spacer_10mm_4_RIGID/RConn3
  Cylindrical55/RConn1 -- QRM102_Frame_Spacer_10mm_32_RIGID/LConn1
  Cylindrical56/LConn1 -- QRM102_Frame_Spacer_10mm_32_RIGID/RConn1
  Cylindrical56/RConn1 -- QRM005_Top_Frame_Ring_1_RIGID/LConn1
  QRM004_Bottom_Frame_Ring_1_RIGID/LConn1 -- Transform/RConn1
  Transform1/RConn1 -- de_1_RIGID/LConn2
  Cylindrical6/LConn1 -- QRM004_Bottom_Frame_Ring_1_RIGID/RConn7
  Cylindrical6/RConn1 -- QRM102_Frame_Spacer_10mm_5_RIGID/LConn1
  Cylindrical7/LConn1 -- QRM004_Bottom_Frame_Ring_1_RIGID/RConn6
  Cylindrical7/RConn1 -- QRM102_Frame_Spacer_10mm_6_RIGID/LConn1
  QRM004_Bottom_Frame_Ring_1_RIGID/RConn2 -- Revolute8/LConn1
  QRM102_Frame_Spacer_10mm_7_RIGID/LConn1 -- Revolute8/RConn1
  Cylindrical8/LConn1 -- QRM004_Bottom_Frame_Ring_1_RIGID/RConn3
  Cylindrical8/RConn1 -- QRM102_Frame_Spacer_10mm_8_RIGID/LConn2
  QRM004_Bottom_Frame_Ring_1_RIGID/RConn4 -- Revolute9/LConn1
  Cylindrical/LConn1 -- Turnigy_18_11_2000kv_Micro_Brushless_Outrunner_1_RIGID/RConn8
  Revolute9/RConn1 -- socket_head_cap_screw_din_21_RIGID/LConn1
  QRM004_Bottom_Frame_Ring_1_RIGID/RConn1 -- Revolute10/LConn1
  Revolute10/RConn1 -- socket_head_cap_screw_din_22_RIGID/LConn1
  QRM004_Bottom_Frame_Ring_1_RIGID/RConn15 -- Revolute11/LConn1
  Revolute11/RConn1 -- socket_head_cap_screw_din_23_RIGID/LConn1
  QRM004_Bottom_Frame_Ring_1_RIGID/RConn14 -- Revolute12/LConn1
  Revolute12/RConn1 -- socket_head_cap_screw_din_24_RIGID/LConn1
  QRM004_Bottom_Frame_Ring_1_RIGID/RConn13 -- Revolute13/LConn1
  Revolute13/RConn1 -- socket_head_cap_screw_din_25_RIGID/LConn1
  QRM004_Bottom_Frame_Ring_1_RIGID/RConn12 -- Revolute14/LConn1
  Cylindrical/RConn1 -- x5x3L_Propeller_3_RIGID/LConn1
  Revolute14/RConn1 -- socket_head_cap_screw_din_26_RIGID/LConn1
  QRM004_Bottom_Frame_Ring_1_RIGID/RConn11 -- Revolute15/LConn1
  Revolute15/RConn1 -- socket_head_cap_screw_din_27_RIGID/LConn1
  QRM004_Bottom_Frame_Ring_1_RIGID/RConn10 -- Revolute16/LConn1
  Revolute16/RConn1 -- socket_head_cap_screw_din_28_RIGID/LConn1
  QRM006_Electronic_Cover_1_RIGID/RConn5 -- Revolute17/LConn1
  Revolute17/RConn1 -- socket_head_cap_screw_din_1_RIGID/LConn1
  QRM006_Electronic_Cover_1_RIGID/RConn4 -- Revolute18/LConn1
  Revolute18/RConn1 -- socket_head_cap_screw_din_2_RIGID/LConn1
  QRM006_Electronic_Cover_1_RIGID/RConn3 -- Revolute19/LConn1
  Planar1/LConn1 -- x5x3L_Propeller_4_RIGID/RConn1
  Revolute19/RConn1 -- socket_head_cap_screw_din_3_RIGID/LConn1
  QRM006_Electronic_Cover_1_RIGID/RConn2 -- Revolute20/LConn1
  Revolute20/RConn1 -- socket_head_cap_screw_din_4_RIGID/LConn1
  QRM003_Battery_Tray_1_RIGID/RConn5 -- Revolute21/LConn1
  Revolute21/RConn1 -- socket_head_cap_screw_din_5_RIGID/LConn1
  QRM003_Battery_Tray_1_RIGID/RConn4 -- Revolute22/LConn1
  Revolute22/RConn1 -- socket_head_cap_screw_din_6_RIGID/LConn1
  QRM003_Battery_Tray_1_RIGID/RConn3 -- Revolute23/LConn1
  Revolute23/RConn1 -- socket_head_cap_screw_din_9_RIGID/LConn1
  Prismatic2/LConn1 -- QRM006_Electronic_Cover_1_RIGID/RConn1
  Planar1/RConn1 -- x5x3R_Propeller_2_RIGID/LConn3
  Prismatic2/RConn1 -- Spektrum_AR6110_1_RIGID/LConn1
  Planar2/LConn1 -- QRM102_Frame_Spacer_10mm_1_RIGID/RConn3
  Planar2/RConn1 -- QRM102_Frame_Spacer_10mm_6_RIGID/LConn2
  Planar3/LConn1 -- QRM102_Frame_Spacer_10mm_1_RIGID/RConn2
  Planar3/RConn1 -- QRM102_Frame_Spacer_10mm_8_RIGID/LConn3
  Planar4/LConn1 -- QRM102_Frame_Spacer_10mm_2_RIGID/RConn3
  Planar4/RConn1 -- QRM102_Frame_Spacer_10mm_3_RIGID/LConn1
  Planar5/LConn1 -- QRM102_Frame_Spacer_10mm_2_RIGID/RConn2
  Planar5/RConn1 -- QRM102_Frame_Spacer_10mm_6_RIGID/LConn3
  Planar6/LConn1 -- QRM102_Frame_Spacer_10mm_3_RIGID/RConn2
  Cylindrical1/LConn1 -- Turnigy_18_11_2000kv_Micro_Brushless_Outrunner_3_RIGID/RConn5
  Planar6/RConn1 -- QRM102_Frame_Spacer_10mm_4_RIGID/LConn2
  Planar7/LConn1 -- QRM102_Frame_Spacer_10mm_5_RIGID/RConn2
  Planar7/RConn1 -- QRM102_Frame_Spacer_10mm_7_RIGID/LConn2
  Planar8/LConn1 -- QRM102_Frame_Spacer_10mm_7_RIGID/RConn2
  Planar8/RConn1 -- QRM102_Frame_Spacer_10mm_8_RIGID/LConn1
  Revolute24/LConn1 -- Turnigy_18_11_2000kv_Micro_Brushless_Outrunner_1_RIGID/RConn7
  Revolute24/RConn1 -- hex_nut_style_1_gradeab_din_1_RIGID/LConn1
  Revolute25/LConn1 -- Turnigy_18_11_2000kv_Micro_Brushless_Outrunner_1_RIGID/RConn6
  Revolute25/RConn1 -- hex_nut_style_1_gradeab_din_2_RIGID/LConn1
  Revolute26/LConn1 -- Turnigy_18_11_2000kv_Micro_Brushless_Outrunner_1_RIGID/RConn5
